simulink model "maze_runner"  (R2025a)
settings: Solver=VariableStepAuto  StartTime=0.0  StopTime=2  RelTol=1e-3
libraries: mmuct_lib x1
settings Model: Creator=llamalulu  LastModifiedBy=llamalulu

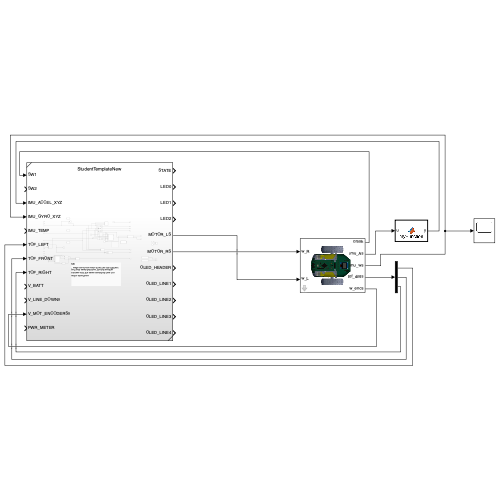
[thumbnail: Simulink's stored preview of the top-level diagram]
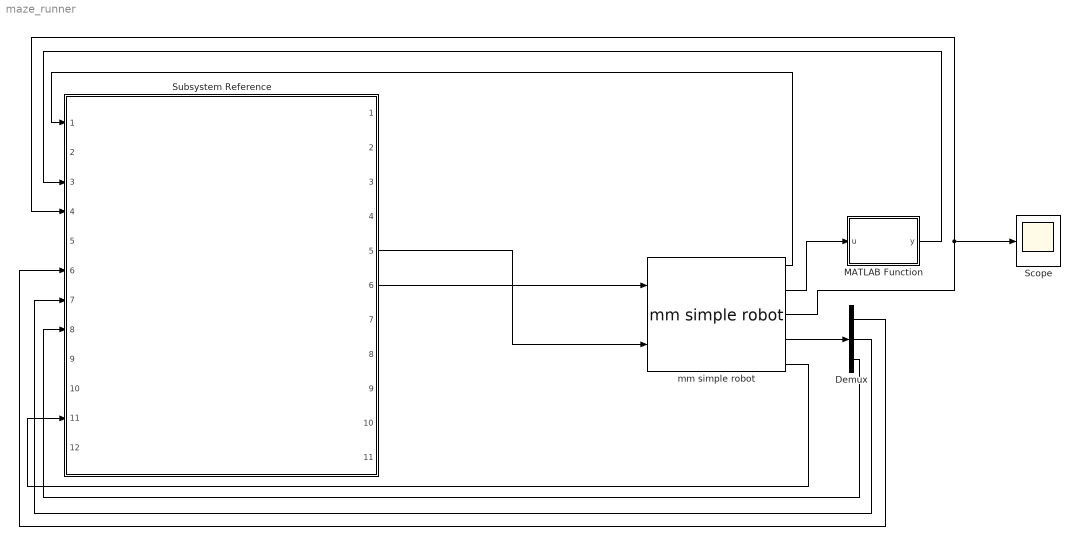
== system maze_runner ==
  Demux : Demux  Outputs=3
  MATLAB Function : MATLAB Function  TreatAsAtomicUnit=on
  Scope : Scope
      settings: DataLoggingVariableName=ScopeData4
  Subsystem Reference : Subsystem  ReferencedSubsystem=StudentTemplateNew
  mm simple robot : mmuct_lib/mm simple robot  simstruct=simstruct  x0=0.1  y0=0.1  theta0=0
  wires:
  mm simple robot/4 -> Demux/1
  Demux/1 -> Subsystem Reference/6
  Demux/2 -> Subsystem Reference/7
  Demux/3 -> Subsystem Reference/8
  Subsystem Reference/6 -> mm simple robot/1
  Subsystem Reference/5 -> mm simple robot/2
  mm simple robot/1 -> Subsystem Reference/1
  mm simple robot/2 -> MATLAB Function/1(u)
  MATLAB Function/1(y) -> Subsystem Reference/3
  mm simple robot/3 -> Subsystem Reference/4, Scope/1
  mm simple robot/5 -> Subsystem Reference/11

== matlab function maze_runner/MATLAB Function ==
  data: u input; y output
function y = myFunction(u)
    %#codegen
    % Ensure the output is a column vector of size [3, 1]
    y = zeros(3, 1); % Explicitly define output size as [3, 1]

    % Example logic: Fill the output based on the input
    if length(u) >= 3
        y(1) = u(1); % Assign first element from input
        y(2) = u(2); % Assign second element from input
        y(3) = u(3); % Assign third element from input
    else
        % Handle cases where input is less than 3 elements
        y(1:length(u)) = u; % Assign available elements
    end
end
